simulink library "UserBlocks"  (R2014a)
settings: Solver=ode45  SolverMode=SingleTasking  StartTime=0.0  StopTime=10.0  RelTol=1e-3
values from neighbouring files (symbols this model uses):
  a = param.a    [DSC_Control_Analysis.m]    (also in DSC_Control_Analysis_Exp.m; DSC_Speed_Control_Analysis.m; EmpiricalTireCurves.m = 1.35; FFW_Fx.m = sqrt(curvature/(2*clothoidLength)))
  b = 1.15    [EmpiricalTireCurves.m]
  Cfls = Cfl    [EC_params_nissan.m]
  Crls = Crl    [EC_params_nissan.m]
  d0 = CSTR.d0    [Ext_MPCPara.m]
  freq = Fs/2*linspace(0,1,NFFT/2)    [AACplottingcode.m]    (also in If_alpha_tp_observer.m; If_alpha_tp_observer_for_c_code.m; If_alpha_tp_observer_shoreline.m)
  Iz = param.Iz    [DSC_Control_Analysis.m]    (also in DSC_Control_Analysis_Exp.m; DSC_Speed_Control_Analysis.m; EmpiricalTireCurves.m = 1300)
  K = 10    [EC_params_nissan.m]
  Ks = -10    [EC_params_nissan.m]
  Ksl = -10    [EC_params_nissan.m]
  Kt = 40000    [EC_params_nissan.m]
  Ku = -40000    [EC_params_nissan.m]
  m = 1724    [EmpiricalTireCurves.m]
  mu_s = mu_p    (= 0.6)    [EC_params_nissan.m]    (also in EmpiricalTireCurves.m = 0.55)
  Ns = 10    [EC_params_nissan.m]
  num = num+MTnum(m)    [Build_MtMuMy.m]
  q = 1    [EC_params_nissan.m]
  Taoh = CSTR.Taoh    [Ext_MPCPara.m]
  Ts = 0.002    [DSC_Control_Analysis.m]    (also in DSC_Control_Analysis_Exp.m; DSC_Speed_Control_Analysis.m; EC_params_nissan.m; Ext_MPCPara.m = SSD.Ts)
undefined symbols (not defined in the file or in its folder): acceAmp, ack, alphaFrontSteeringLimit, alphaFrontTable, bit, c, Cfl, Crl, CSTR, dden, deltaPsiDotGain, deltDist, den, denafilt, dnum, elaDotGain, filtera, filterb, frontAlphaLookup, frontForceLookup, FuelStartCalTime, FyFtable, gpsins, h, h_roll, hal_filter_den, hal_filter_num, hwx, hwy5, initAcce, initSpeed, isDriverNoise, lkparams, mapDataFull, mapMatchingParams, maxFrontForce, maxNumSegs, mdPtrs, numafilt, param, rearAlphaLookup, rfl, rfr, rrl, rrr, sglu, SIMP, simuCond, slimFxl, slimFxu, sliml, slimMll, slimMlr, slimMul, slimMur, slimu, sr, SSD, Standard, steering_limit ... (+7)
libraries: simulink x28, slrtlib x18, UserBlocks x6, slrtsoftinglib x6, MickLibBlocks x1, DriftControllerLibrary x1
(part 1 of 6)
settings Model: Creator=ddl  LastModifiedBy=cbeal

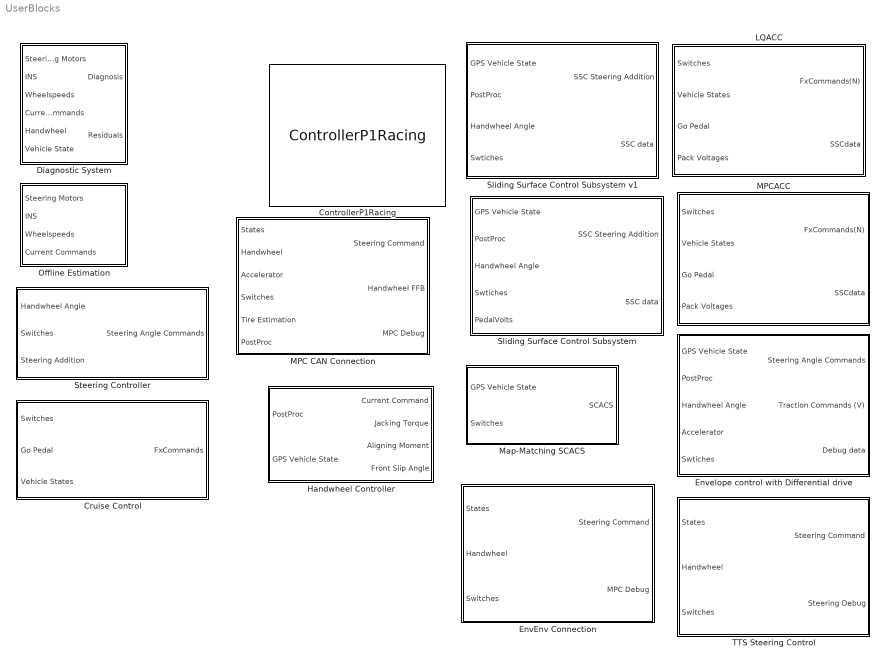
== system UserBlocks ==
  ControllerP1Racing : MickLibBlocks/ControllerP1Racing  SystemSampleTime=-1
  Cruise Control : Subsystem
      mask init:
      | CruiseControl
  Diagnostic System : Subsystem
  EnvEnv Connection : Subsystem
      mask init:
      | p1_params;
      | SteeringController;
  Envelope control with Differential drive : Subsystem
      mask init:
      | % get P1 parameters
      | p1_params;
      | 
      | % get params to filter handwheel angle
      | SteeringController;
      | 
      | Ts=0.002;
  Handwheel Controller : Subsystem
      mask init:
      | hw_lookuptable;
      | p1_params;
  LQACC : Subsystem
      mask init:
      | CruiseControl;
      | p1_params;
      | Main_MPC_MTCACC1;
  MPC CAN Connection : Subsystem
      mask init:
      | p1_params;
      | SteeringController;
  MPCACC : Subsystem
      mask init:
      | Ts = .002;
      | CruiseControl;
      | p1_params;
      | %Para_CYL52;
      | 
      | %self_ChangeDir;
      | Main_MPC_MTCACC1;
      | 
      | mpc_params;
      | LL_CtrlObj;
      | Ext_MPCpara;
      | Proc_RT_para;
  Map-Matching SCACS : Subsystem
  Offline Estimation : Subsystem
  Sliding Surface Control Subsystem : Subsystem
      mask init:
      | % get SSC parameters
      | p1_params;
      | slidingsurface_params;
      | 
      | % get params to filter handwheel angle
      | SteeringController;
  Sliding Surface Control Subsystem v1 : Subsystem
      mask init:
      | % get SSC parameters
      | p1_params;
      | slidingsurface_params;
      | 
      | % get params to filter handwheel angle
      | SteeringController;
  Steering Controller : Subsystem
      mask init:
      | p1_params;
      | SteeringController;
  TTS Steering Control : Subsystem
      mask init:
      | p1_params;
      | SteeringController;

== system UserBlocks/Cruise Control ==
  Switches : Inport
  Go Pedal : Inport  Port=2
  Vehicle States : Inport  Port=3
  Bus Selector : BusSelector  OutputSignals=Vx
  Bus Selector1 : BusSelector  OutputSignals=Cruise Control Switch,Brake Pedal Signal
  ConvertVolt2Force : Subsystem
  Enable Logic : Subsystem
  Gain : Gain
  Mux1 : Mux  Inputs=2
  Pedal Latch : Subsystem  TreatAsAtomicUnit=on
  Quantizer : Quantizer  QuantizationInterval=5
  Speed Latch : Subsystem  TreatAsAtomicUnit=on
  Sum : Sum  Inputs=-+|
  Sum1 : Sum  Inputs=|++
  Switch : Switch  Threshold=.5
  FxCommands : Outport
  wires:
  Go Pedal/1 -> Pedal Latch/1(In1), Switch/3
  Switches/1 -> Bus Selector1/1
  Sum/1 -> Gain/1
  Enable Logic/1(Enable) -> Switch/2
  Mux1/1 -> ConvertVolt2Force/1(VoltDesired)
  Switch/1 -> Mux1/2, Mux1/1
  Speed Latch/1(Out1) -> Quantizer/1
  Gain/1 -> Sum1/1
  Sum1/1 -> Switch/1
  Pedal Latch/1(Out1) -> Sum1/2
  Bus Selector1/1 -> Enable Logic/1(Cruise Control), Pedal Latch/Trigger, Speed Latch/Trigger  "<Cruise Control Switch>"
  Bus Selector1/2 -> Enable Logic/2(Brake Pedal)  "<Brake Pedal Signal>"
  Quantizer/1 -> Sum/2
  Bus Selector/1 -> Speed Latch/1(In1), Sum/1  "<Vx>"
  Vehicle States/1 -> Bus Selector/1
  ConvertVolt2Force/1(TorqueDesired) -> FxCommands/1

== system UserBlocks/Diagnostic System ==
  Steering Motors : Inport
  INS : Inport  Port=2
  Wheelspeeds : Inport  Port=3
  Current Commands : Inport  Port=4
  Handwheel : Inport  Port=5
  Vehicle State : Inport  Port=6
  Bus Selector : BusSelector  OutputSignals=Roll Angle
  Bus Selector1 : BusSelector  OutputSignals=Primary
  Bus Selector2 : BusSelector  OutputSignals=Front Wheel Speeds
  Detection : Subsystem
      mask Display: disp('')
  Filtering : Subsystem
      mask Display: disp('')
  Isolation : Subsystem
      mask Display: disp('')
  Residual Generation : Subsystem
  Diagnosis : Outport
  Residuals : Outport  Port=2
  wires:
  Steering Motors/1 -> Residual Generation/1(Steering Motors)
  INS/1 -> Residual Generation/2(INS)
  Residual Generation/1(Residuals) -> Filtering/1(Residuals)
  Detection/1(Boolean Residuals) -> Isolation/1(Boolean Residuals)
  Current Commands/1 -> Residual Generation/4(Current Commands)
  Wheelspeeds/1 -> Bus Selector2/1
  Isolation/1(Diagnosis) -> Diagnosis/1
  Filtering/1(Filtered Residuals) -> Detection/1(Filtered Residuals), Residuals/1
  Vehicle State/1 -> Bus Selector/1
  Bus Selector/1 -> Residual Generation/6(Roll Angle)  "<Roll Angle>"
  Handwheel/1 -> Bus Selector1/1
  Bus Selector1/1 -> Residual Generation/5(Handwheel)  "<Primary>"
  Bus Selector2/1 -> Residual Generation/3(Wheelspeeds)  "<Front Wheel Speeds>"

== system UserBlocks/EnvEnv Connection ==
  States : Inport
  Handwheel : Inport  Port=2
  Switches : Inport  Port=3
  Ackermann Correction : Subsystem
  Bus Selector2 : BusSelector  OutputSignals=Primary
  Bus Selector4 : BusSelector  OutputSignals=Auto-Steer Switch
  Compute delta Steer : Subsystem
  Mux6 : Mux  Inputs=2
  SW Steering Limit : Saturate  UpperLimit=steering_limit*pi/180  LowerLimit=-steering_limit*pi/180
  SW Steering Limit1 : Saturate  UpperLimit=steering_limit*pi/180  LowerLimit=-steering_limit*pi/180
  Subsystem : Subsystem
  Sum : Sum  Inputs=|++
  Sum1 : Sum  Inputs=|++
  delta offset : Constant  Value=0*pi/180
  Steering Command : Outport
  MPC Debug : Outport  Port=2
  wires:
  delta offset/1 -> Sum1/2
  Sum1/1 -> SW Steering Limit/1
  Sum/1 -> Sum1/1
  Compute delta Steer/2(MPC Debug) -> MPC Debug/1
  States/1 -> Compute delta Steer/1(States)
  Compute delta Steer/1(delta Steering Command) -> Sum/2
  SW Steering Limit1/1 -> Compute delta Steer/2(driver Steer Cmd), Sum/1
  Bus Selector4/1 -> Subsystem/2(Switches)  "<Auto-Steer Switch>"
  Bus Selector2/1 -> Subsystem/1(Handwheel)  "<Primary>"
  Switches/1 -> Compute delta Steer/3(Switches), Bus Selector4/1
  Handwheel/1 -> Bus Selector2/1
  Subsystem/1(Steering Output) -> SW Steering Limit1/1
  Ackermann Correction/2(R Steer Angle) -> Mux6/2
  Ackermann Correction/1(L Steer Angle) -> Mux6/1
  SW Steering Limit/1 -> Ackermann Correction/1(Ackermann Angle)
  Mux6/1 -> Steering Command/1

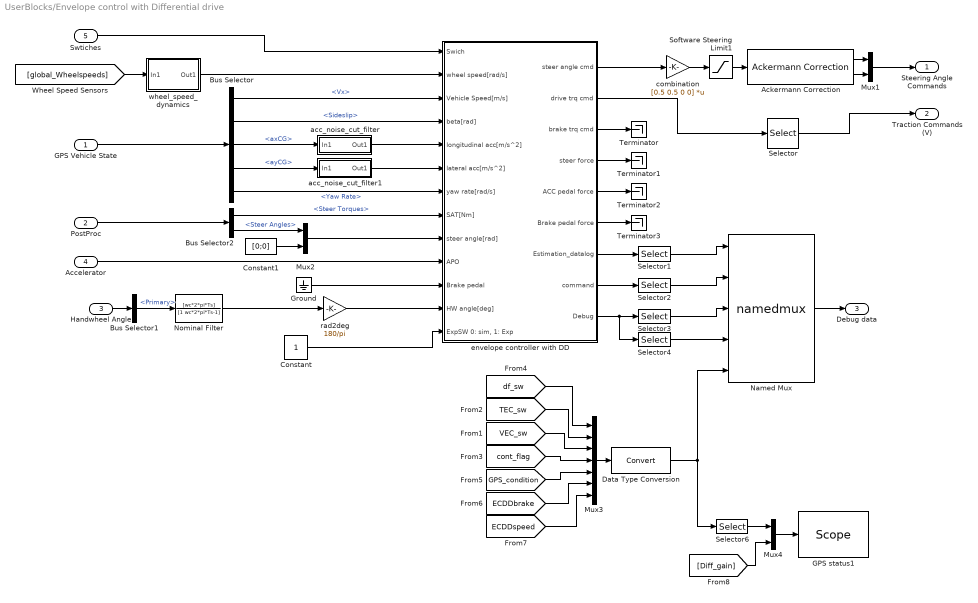
== system UserBlocks/Envelope control with Differential drive ==
  GPS Vehicle State : Inport
  PostProc : Inport  Port=2
  Handwheel Angle : Inport  Port=3
  Accelerator : Inport  Port=4
  Swtiches : Inport  Port=5
  Ackermann Correction : UserBlocks/Steering Controller/Ackermann Correction
  Bus Selector : BusSelector  OutputSignals=Vx,Sideslip,axCG,ayCG,Yaw Rate
  Bus Selector1 : BusSelector  OutputSignals=Primary
  Bus Selector2 : BusSelector  OutputSignals=Steer Torques,Steer Angles
  Constant : Constant
  Constant1 : Constant  Value=[0;0]
  Data Type Conversion : DataTypeConversion
  GPS status1 : slrtlib/Displays and Logging/Scope   scopeno=2  scopetype=Target  autostart=on  viewmode=Numerical  formatstr='%15.6f'  grid=on  ylimits=[-10,10]  nosamples=round(1/Ts)  noprepostsamples=0  interleave=1  triggermode=FreeRun  triggersignal=1  trigsignalfromport=off  triggerlevel=0.0  triggerslope=Either  triggerscope=1  triggersample=0  filename=data.dat  mode=Lazy  writesize=512  autorestart=off  dynamicfilemode=off  maxwritefilesize=512*1024^2
  Ground : Ground
  Mux1 : Mux  Inputs=2
  Mux2 : Mux  Inputs=2
  Mux3 : Mux  Inputs=7
  Mux4 : Mux  Inputs=2
  Named Mux : S-Function  FunctionName=namedmux  Parameters=inputcount,inputsizes  EnableBusSupport=off  mask{fname=datadescTCS}
      mask prompts: fname "Data description function name"
      mask help:
      | Combines input signals into a single output vector, according to a structure that provides the names and sizes of each signal.
      |
      | The parameter below should be set to the name of a function which returns a 1xN structure array, where N is the number of input signals.  The structure should contain fields "size" which specifies the width of the input signal, and "name" which specifies its name.
      mask init:
      | desc=eval(fname);
      | %if(class(desc)~='cell')
      | %	error('Incorrect description');
      | %end
      | inputcount=length(desc);
      | if((inputcount<1)|(inputcount>50))
      | 	error('Inappropriate number of inputs.');
      | end
      | 
      | inputsizes=[desc.size];
      | 
      | x=min(inputcount*ones(1,50),1:50);
      mask Display:
      | port_label('input',x(1),desc(x(1)).name);
      | port_label('input',x(2),desc(x(2)).name);
      | port_label('input',x(3),desc(x(3)).name);
      | port_label('input',x(4),desc(x(4)).name);
      | port_label('input',x(5),desc(x(5)).name);
      | port_label('input',x(6),desc(x(6)).name);
      | port_label('input',x(7),desc(x(7)).name);
      | port_label('input',x(8),desc(x(8)).name);
      | port_label('input',x(9),desc(x(9)).name);
      | port_label('input',x(10),desc(x(10)).name);
      | port_label('input',x(11),desc(x(11)).name);
      | port_label('input',x(12),desc(x(12)).name);
      | port_label('input',x(13),desc(x(13)).name);
      | port_label('input',x(14),desc(x(14)).name);
      | port_label('input',x(15),desc(x(15)).name);
      | port_label('input',x(16),desc(x(16)).name);
      | port_label('input',x(17),desc(x(17)).name);
      | port_label('input',x(18),desc(x(18)).name);
      | port_label('input',x(19),desc(x(19)).name);
      | port_label('input',x(20),desc(x(20)).name);
      | port_label('input',x(21),desc(x(21)).name);
      | port_label('input',x(22),desc(x(22)).name);
      | port_label('input',x(23),desc(x(23)).name);
      | port_label('input',x(24),desc(x(24)).name);
      | port_label('input',x(25),desc(x(25)).name);
      | port_label('input',x(26),desc(x(26)).name);
      | port_label('input',x(27),desc(x(27)).name);
      | port_label('input',x(28),desc(x(28)).name);
      | port_label('input',x(29),desc(x(29)).name);
      | port_label('input',x(30),desc(x(30)).name);
  Nominal Filter : DiscreteFilter  Numerator=[wc*2*pi*Ts]  Denominator=[1 wc*2*pi*Ts-1]  SampleTime=Ts
  Selector : Selector  InputPortWidth=4  Indices=[4 3]
  Selector1 : Selector  InputPortWidth=17  Indices=[1:4]
  Selector2 : Selector  InputPortWidth=9  Indices=[7:9]
  Selector3 : Selector  InputPortWidth=19  Indices=[1:8]
  Selector4 : Selector  InputPortWidth=19  Indices=[9,11:19]
  Selector6 : Selector  InputPortWidth=7  Indices=[4:7]
  Software Steering Limit1 : Saturate  UpperLimit=steering_limit*pi/180  LowerLimit=-steering_limit*pi/180
  Terminator{,1..3} (4 alike) : Terminator
  acc_noise_cut_filter : Subsystem
      mask init:
      | [numafilt,denafilt]=butter(2,0.02);
  acc_noise_cut_filter1 : Subsystem
      mask init:
      | [numafilt,denafilt]=butter(2,0.02);
  combination : Gain  Gain=[0.5 0.5 0 0]  Multiplication=Matrix(K*u)
  envelope controller with DD : Subsystem
      mask init:
      | p1_params
  rad2deg : Gain  Gain=180/pi
  wheel_speed_dynamics : Subsystem
      mask init:
      | p1_params
      | EC_params_nissan
      | [filterb,filtera]=butter(2,0.03);
  Steering Angle Commands : Outport
  Traction Commands (V) : Outport  Port=2
  Debug data : Outport  Port=3
  wires:
  [Diff_gain] -> Mux4/2
  Mux4/1 -> GPS status1/1
  Selector6/1 -> Mux4/1
  [ECDDspeed] -> Mux3/7
  [ECDDbrake] -> Mux3/6
  [GPS_condition] -> Mux3/5
  [cont_flag] -> Mux3/4
  [VEC_sw] -> Mux3/3
  [TEC_sw] -> Mux3/2
  [df_sw] -> Mux3/1
  Selector4/1 -> Named Mux/4
  acc_noise_cut_filter1/1(Out1) -> envelope controller with DD/6(lateral acc[m/s^2])
  acc_noise_cut_filter/1(Out1) -> envelope controller with DD/5(longitudinal acc[m/s^2])
  Data Type Conversion/1 -> Named Mux/5, Selector6/1
  Handwheel Angle/1 -> Bus Selector1/1
  Ground/1 -> envelope controller with DD/11(Brake pedal)
  Mux2/1 -> envelope controller with DD/9(steer angle[rad])
  Software Steering Limit1/1 -> Ackermann Correction/1
  Ackermann Correction/1 -> Mux1/1
  Ackermann Correction/2 -> Mux1/2
  Mux1/1 -> Steering Angle Commands/1
  combination/1 -> Software Steering Limit1/1
  Selector/1 -> Traction Commands (V)/1
  envelope controller with DD/3(brake trq cmd) -> Terminator/1
  envelope controller with DD/4(steer force) -> Terminator1/1
  envelope controller with DD/5(ACC pedal force) -> Terminator2/1
  envelope controller with DD/6(Brake pedal force) -> Terminator3/1
  envelope controller with DD/7(Estimation_datalog) -> Selector1/1
  envelope controller with DD/2(drive trq cmd) -> Selector/1
  envelope controller with DD/8(command) -> Selector2/1
  envelope controller with DD/9(Debug) -> Selector3/1, Selector4/1
  Selector1/1 -> Named Mux/1
  Selector2/1 -> Named Mux/2
  Selector3/1 -> Named Mux/3
  Named Mux/1 -> Debug data/1
  Bus Selector1/1 -> Nominal Filter/1  "<Primary>"
  Nominal Filter/1 -> rad2deg/1
  rad2deg/1 -> envelope controller with DD/12(HW angle[deg])
  Constant/1 -> envelope controller with DD/13("ExpSW 0: sim, 1: Exp")
  GPS Vehicle State/1 -> Bus Selector/1
  PostProc/1 -> Bus Selector2/1
  Bus Selector2/1 -> envelope controller with DD/8(SAT[Nm])  "<Steer Torques>"
  Bus Selector2/2 -> Mux2/1  "<Steer Angles>"
  Constant1/1 -> Mux2/2
  Accelerator/1 -> envelope controller with DD/10(APO)
  Bus Selector/1 -> envelope controller with DD/3(Vehicle Speed[m/s])  "<Vx>"
  Bus Selector/5 -> envelope controller with DD/7(yaw rate[rad/s])  "<Yaw Rate>"
  Bus Selector/2 -> envelope controller with DD/4(beta[rad])  "<Sideslip>"
  Bus Selector/3 -> acc_noise_cut_filter/1(In1)  "<axCG>"
  Bus Selector/4 -> acc_noise_cut_filter1/1(In1)  "<ayCG>"
  wheel_speed_dynamics/1(Out1) -> envelope controller with DD/2(wheel speed[rad/s])
  [global_Wheelspeeds] -> wheel_speed_dynamics/1(In1)
  envelope controller with DD/1(steer angle cmd) -> combination/1
  Swtiches/1 -> envelope controller with DD/1(Swich)
  Mux3/1 -> Data Type Conversion/1

== system UserBlocks/Handwheel Controller ==
  note: alpha slide
  note: Fy
  note: pneumatic trail
  note: Simulated Aligning Moment Cmd, max=.7
  note: Simulated Jacking Torque Cmd, max=.25
  note: avg steer angle
  PostProc : Inport
  GPS Vehicle State : Inport  Port=2
  Bus Selector2 : BusSelector  OutputSignals=Composite Steer Angle
  Bus Selector3 : BusSelector  OutputSignals=Vx,Yaw Rate,VyCG
  Gain1 : Gain  Gain=100
  Gain2 : Gain  Gain=1/125
  Gain3 : Gain  Gain=.0008
  Sum : Sum  Inputs=+|+
  T4 : Terminator
  T6 : Terminator
  T7 : Terminator
  estimate_aligningTorque : S-Function  FunctionName=estimate_aligningTorque  Parameters=tp, Cf, Fz_f, tm, b  EnableBusSupport=off
  jacking torque cmd with 0.25 saturation : Lookup  InputValues=hwx.*100  Table=hwy5.*100  OutDataTypeStr=float('double')  SaturateOnIntegerOverflow=on
  Current Command : Outport
  Jacking Torque : Outport  Port=2
  Aligning Moment : Outport  Port=3
  Front Slip Angle : Outport  Port=4
  wires:
  estimate_aligningTorque/5 -> Front Slip Angle/1  "alpha_f"
  Bus Selector3/3 -> estimate_aligningTorque/4  "<VyCG>"
  Bus Selector3/2 -> estimate_aligningTorque/3  "<Yaw Rate>"
  Bus Selector3/1 -> estimate_aligningTorque/2  "<Vx>"
  GPS Vehicle State/1 -> Bus Selector3/1
  Sum/1 -> Current Command/1
  Gain3/1 -> Aligning Moment/1, Sum/2  "Align Mom Cmd"
  estimate_aligningTorque/1 -> Gain3/1
  estimate_aligningTorque/4 -> T7/1
  estimate_aligningTorque/3 -> T6/1
  estimate_aligningTorque/2 -> T4/1
  Bus Selector2/1 -> estimate_aligningTorque/1, Gain1/1  "<Composite Steer Angle>"
  Gain2/1 -> Jacking Torque/1, Sum/1  "Jack Torque Cmd"
  jacking torque cmd with 0.25 saturation/1 -> Gain2/1
  Gain1/1 -> jacking torque cmd with 0.25 saturation/1
  PostProc/1 -> Bus Selector2/1

== system UserBlocks/LQACC ==
  Switches : Inport
  Vehicle States : Inport  Port=2
  Go Pedal : Inport  Port=3
  Pack Voltages : Inport  Port=4
  Bus Creator : BusCreator  Inputs=10
  Bus Selector : BusSelector  OutputSignals=Traction
  PIDACC : Subsystem  AncestorBlock=UserBlocks/Cruise Control
      mask init:
      | CruiseControl;
      | p1_params;
      | Main_MPC_MTCACC1;
  FxCommands(N) : Outport
  SSCdata : Outport  Port=2
  wires:
  PIDACC/10(vehACCE) -> Bus Creator/10
  PIDACC/9(relVEL) -> Bus Creator/9
  PIDACC/8(distErr) -> Bus Creator/8
  PIDACC/7(desAcce(m/s2)) -> Bus Creator/6
  Pack Voltages/1 -> Bus Selector/1
  Bus Creator/1 -> SSCdata/1
  Switches/1 -> PIDACC/1(Switches)
  Vehicle States/1 -> PIDACC/2(Vehicle States)
  Go Pedal/1 -> PIDACC/3(Go Pedal1)
  Bus Selector/1 -> Bus Creator/7  "<Traction>"
  PIDACC/1(FxCommands(N)) -> FxCommands(N)/1
  PIDACC/2(PreAcce(m/s2)) -> Bus Creator/1
  PIDACC/3(PreSpeec(m/s)) -> Bus Creator/2
  PIDACC/4(epsilon) -> Bus Creator/3
  PIDACC/5(DesDist(m)) -> Bus Creator/4
  PIDACC/6(ActDist(m)) -> Bus Creator/5

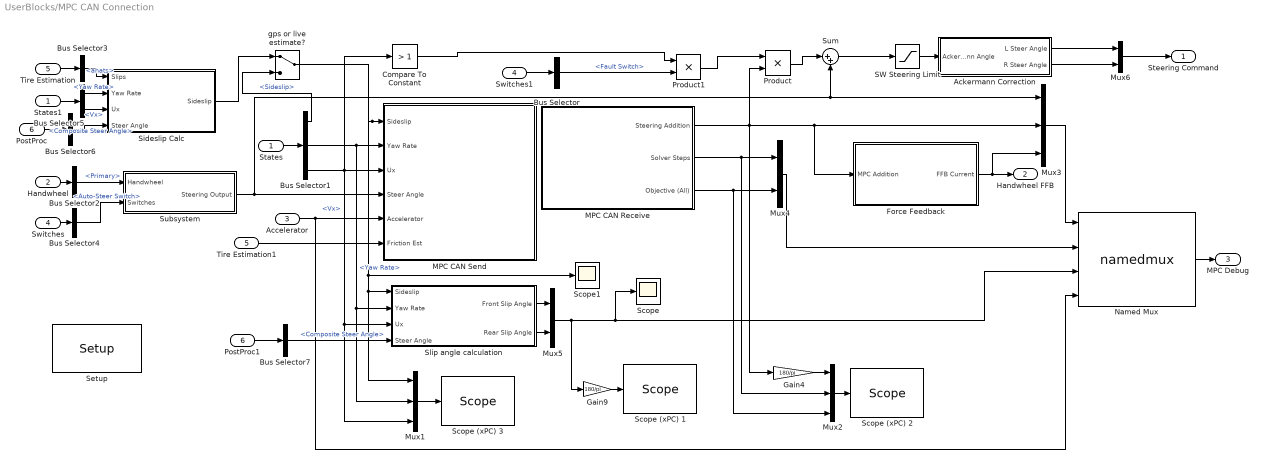
== system UserBlocks/MPC CAN Connection ==
  States : Inport
  Handwheel : Inport  Port=2
  Accelerator : Inport  Port=3
  Switches : Inport  Port=4
  Tire Estimation : Inport  Port=5
  PostProc : Inport  Port=6
  Ackermann Correction : Subsystem
  Bus Selector : BusSelector  OutputSignals=Fault Switch
  Bus Selector1 : BusSelector  OutputSignals=Sideslip,Yaw Rate,Vx
  Bus Selector2 : BusSelector  OutputSignals=Primary
  Bus Selector3 : BusSelector  OutputSignals=ahats
  Bus Selector4 : BusSelector  OutputSignals=Auto-Steer Switch
  Bus Selector5 : BusSelector  OutputSignals=Yaw Rate,Vx
  Bus Selector6 : BusSelector  OutputSignals=Composite Steer Angle
  Bus Selector7 : BusSelector  OutputSignals=Composite Steer Angle
  Compare To Constant : simulink/Logic and Bit Operations/Compare To Constant  relop=>  const=1  OutDataTypeStr=uint8  ZeroCross=off
  Force Feedback : Subsystem  mask{steer_gain=0, current_limit=0}
      mask prompts: steer_gain "FFB Gain (A/rad)"; current_limit "Current Limit (A)"
  Gain4 : Gain  Gain=180/pi
  Gain9 : Gain  Gain=180/pi
  MPC CAN Receive : Subsystem
  MPC CAN Send : Subsystem
  Mux1 : Mux  Inputs=3
  Mux2 : Mux  Inputs=3
  Mux3 : Mux  Inputs=3
  Mux4 : Mux  Inputs=2
  Mux5 : Mux  Inputs=2
  Mux6 : Mux  Inputs=2
  Named Mux : S-Function  FunctionName=namedmux  Parameters=inputcount,inputsizes  EnableBusSupport=off  mask{fname=datadescMPCEnv}
      mask prompts: fname "Data description function name"
      mask help:
      | Combines input signals into a single output vector, according to a structure that provides the names and sizes of each signal.
      |
      | The parameter below should be set to the name of a function which returns a 1xN structure array, where N is the number of input signals.  The structure should contain fields "size" which specifies the width of the input signal, and "name" which specifies its name.
      mask init: same as UserBlocks/Envelope control with Differential drive/Named Mux
      mask Display:
      | port_label('input',x(1),desc(x(1)).name);
      | port_label('input',x(2),desc(x(2)).name);
      | port_label('input',x(3),desc(x(3)).name);
      | port_label('input',x(4),desc(x(4)).name);
      | port_label('input',x(5),desc(x(5)).name);
      | port_label('input',x(6),desc(x(6)).name);
      | port_label('input',x(7),desc(x(7)).name);
      | port_label('input',x(8),desc(x(8)).name);
      | port_label('input',x(9),desc(x(9)).name);
      | port_label('input',x(10),desc(x(10)).name);
      | port_label('input',x(11),desc(x(11)).name);
      | port_label('input',x(12),desc(x(12)).name);
      | port_label('input',x(13),desc(x(13)).name);
      | port_label('input',x(14),desc(x(14)).name);
      | port_label('input',x(15),desc(x(15)).name);
      | port_label('input',x(16),desc(x(16)).name);
      | port_label('input',x(17),desc(x(17)).name);
      | port_label('input',x(18),desc(x(18)).name);
      | port_label('input',x(19),desc(x(19)).name);
      | port_label('input',x(20),desc(x(20)).name);
      | port_label('input',x(21),desc(x(21)).name);
      | port_label('input',x(22),desc(x(22)).name);
      | port_label('input',x(23),desc(x(23)).name);
      | port_label('input',x(24),desc(x(24)).name);
      | port_label('input',x(25),desc(x(25)).name);
      | port_label('input',x(26),desc(x(26)).name);
      | port_label('input',x(27),desc(x(27)).name);
      | port_label('input',x(28),desc(x(28)).name);
      | port_label('input',x(29),desc(x(29)).name);
      | port_label('input',x(30),desc(x(30)).name);
  PostProc1 : InportShadow  Port=6
  Product : Product  RndMeth=Zero
  Product1 : Product  RndMeth=Zero
  SW Steering Limit : Saturate  UpperLimit=steering_limit*pi/180  LowerLimit=-steering_limit*pi/180
  Scope : Scope
  Scope (xPC) 1 : slrtlib/Displays and Logging/Scope   scopeno=3  scopetype=Target  autostart=on  viewmode=Graphical rolling  formatstr='%15.6f'  grid=on  ylimits=[-10,10]  nosamples=50  noprepostsamples=0  interleave=1  triggermode=FreeRun  triggersignal=1  trigsignalfromport=off  triggerlevel=0.0  triggerslope=Either  triggerscope=1  triggersample=0  filename=data.dat  mode=Lazy  writesize=512  autorestart=off  dynamicfilemode=off  maxwritefilesize=512*1024^2
  Scope (xPC) 2 : slrtlib/Displays and Logging/Scope   scopeno=4  scopetype=Target  autostart=on  viewmode=Numerical  formatstr='%15.6f'  grid=on  ylimits=[-1,1]  nosamples=100  noprepostsamples=0  interleave=1  triggermode=FreeRun  triggersignal=1  trigsignalfromport=off  triggerlevel=0.0  triggerslope=Either  triggerscope=1  triggersample=0  filename=data.dat  mode=Lazy  writesize=512  autorestart=off  dynamicfilemode=off  maxwritefilesize=512*1024^2
  Scope (xPC) 3 : slrtlib/Displays and Logging/Scope   scopeno=2  scopetype=Target  autostart=on  viewmode=Numerical  formatstr='%15.6f'  grid=on  ylimits=[-30,30]  nosamples=50  noprepostsamples=0  interleave=1  triggermode=FreeRun  triggersignal=1  trigsignalfromport=off  triggerlevel=0.0  triggerslope=Either  triggerscope=1  triggersample=0  filename=data.dat  mode=Lazy  writesize=512  autorestart=off  dynamicfilemode=off  maxwritefilesize=512*1024^2
  Scope1 : Scope
  "Setup " : slrtsoftinglib/CAN-AC2-104 SJA 1000/Setup   board=1  can1Baudrate=500 kBaud  can1UserBR=[1,1,4,3]  can2Baudrate=500 kBaud  can2UserBR=[1,1,4,3]  init=[]  term=[]  bus_off_out=off  bus_off_rec=Off  ioBaseAddressL=0x240  memBaseAddressL=0xd0000  intNo=None
  Sideslip Calc : Subsystem  mask{a=1.35, b=1.15}
      mask prompts: a "CG - Front Axle Distance"; b "CG - Rear Axle Distance"
  Slip angle calculation : Subsystem  mask{a=1.35, b=1.15}
      mask prompts: a "CG - Front Axle Distance"; b "CG - Rear Axle Distance"
  States1 : InportShadow
  Subsystem : Subsystem
  Sum : Sum  Inputs=|++
  Switches1 : InportShadow  Port=4
  Tire Estimation1 : InportShadow  Port=5
  gps or live estimate? : ManualSwitch
  Steering Command : Outport
  Handwheel FFB : Outport  Port=2
  MPC Debug : Outport  Port=3
  wires:
  Bus Selector7/1 -> Slip angle calculation/4(Steer Angle)  "<Composite Steer Angle>"
  PostProc1/1 -> Bus Selector7/1
  Bus Selector6/1 -> Sideslip Calc/4(Steer Angle)  "<Composite Steer Angle>"
  PostProc/1 -> Bus Selector6/1
  Bus Selector1/1 -> gps or live estimate?/2  "<Sideslip>"
  gps or live estimate?/1 -> Mux1/1, Slip angle calculation/1(Sideslip), Scope1/1, MPC CAN Send/1(Sideslip)
  Sideslip Calc/1(Sideslip) -> gps or live estimate?/1
  Tire Estimation1/1 -> MPC CAN Send/6(Friction Est)
  Bus Selector5/2 -> Sideslip Calc/3(Ux)  "<Vx>"
  Bus Selector5/1 -> Sideslip Calc/2(Yaw Rate)  "<Yaw Rate>"
  Bus Selector3/1 -> Sideslip Calc/1(Slips)  "<ahats>"
  States1/1 -> Bus Selector5/1
  Tire Estimation/1 -> Bus Selector3/1
  Mux6/1 -> Steering Command/1
  Product1/1 -> Product/1
  Compare To Constant/1 -> Product1/1
  Bus Selector/1 -> Product1/2  "<Fault Switch>"
  Switches1/1 -> Bus Selector/1
  SW Steering Limit/1 -> Ackermann Correction/1(Ackermann Angle)
  Ackermann Correction/1(L Steer Angle) -> Mux6/1
  Ackermann Correction/2(R Steer Angle) -> Mux6/2
  Named Mux/1 -> MPC Debug/1
  Mux5/1 -> Scope/1, Named Mux/3, Gain9/1
  Mux4/1 -> Named Mux/2
  Slip angle calculation/2(Rear Slip Angle) -> Mux5/2
  Slip angle calculation/1(Front Slip Angle) -> Mux5/1
  Gain4/1 -> Mux2/1
  Mux2/1 -> Scope (xPC) 2/1
  States/1 -> Bus Selector1/1
  Bus Selector1/3 -> MPC CAN Send/3(Ux), Slip angle calculation/3(Ux), Mux1/3, Compare To Constant/1  "<Vx>"
  Mux3/1 -> Named Mux/1
  MPC CAN Receive/1(Steering Addition) -> Force Feedback/1(MPC Addition), Mux3/2, Gain4/1, Product/2
  Sum/1 -> SW Steering Limit/1
  Force Feedback/1(FFB Current) -> Handwheel FFB/1, Mux3/3
  Bus Selector1/2 -> MPC CAN Send/2(Yaw Rate), Slip angle calculation/2(Yaw Rate), Mux1/2  "<Yaw Rate>"
  MPC CAN Receive/2(Solver Steps) -> Mux4/1, Mux2/2
  MPC CAN Receive/3(Objective (All)) -> Mux4/2, Mux2/3
  Gain9/1 -> Scope (xPC) 1/1
  Mux1/1 -> Scope (xPC) 3/1
  Accelerator/1 -> Named Mux/4, MPC CAN Send/5(Accelerator)
  Product/1 -> Sum/1
  Subsystem/1(Steering Output) -> Mux3/1, Sum/2, MPC CAN Send/4(Steer Angle)
  Handwheel/1 -> Bus Selector2/1
  Switches/1 -> Bus Selector4/1
  Bus Selector2/1 -> Subsystem/1(Handwheel)  "<Primary>"
  Bus Selector4/1 -> Subsystem/2(Switches)  "<Auto-Steer Switch>"

== system UserBlocks/MPCACC ==
  Switches : Inport
  Vehicle States : Inport  Port=2
  Go Pedal : Inport  Port=3
  Pack Voltages : Inport  Port=4
  Bus Creator : BusCreator  Inputs=10
  Bus Selector : BusSelector  OutputSignals=Traction
  PIDACC : Subsystem  AncestorBlock=UserBlocks/Cruise Control
      mask init:
      | InitModel;
      | CruiseControl;
      | p1_params;
      | Main_MPC_MTCACC1;
  FxCommands(N) : Outport
  SSCdata : Outport  Port=2
  wires:
  PIDACC/6(ActDist(m)) -> Bus Creator/5
  PIDACC/5(DesDist(m)) -> Bus Creator/4
  PIDACC/4(epsilon) -> Bus Creator/3
  PIDACC/3(PreSpeec(m/s)) -> Bus Creator/2
  PIDACC/2(PreAcce(m/s2)) -> Bus Creator/1
  PIDACC/1(FxCommands(N)) -> FxCommands(N)/1
  Bus Selector/1 -> Bus Creator/7  "<Traction>"
  Go Pedal/1 -> PIDACC/3(Go Pedal1)
  Vehicle States/1 -> PIDACC/2(Vehicle States)
  Switches/1 -> PIDACC/1(Switches)
  Bus Creator/1 -> SSCdata/1
  Pack Voltages/1 -> Bus Selector/1
  PIDACC/7(desAcce(m/s2)) -> Bus Creator/6
  PIDACC/8(distErr) -> Bus Creator/8
  PIDACC/9(relVEL) -> Bus Creator/9
  PIDACC/10(vehACCE) -> Bus Creator/10

== system UserBlocks/Map-Matching SCACS ==
  GPS Vehicle State : Inport
  Switches : Inport  Port=2
  Bus Creator : BusCreator  Inputs=6
  Bus Selector : BusSelector  OutputSignals=Pos E,Pos N,Yaw Angle,Vx
  Bus Selector1 : BusSelector  OutputSignals=Auto-Steer Switch
  Constant1 : Constant  Value=pi/2  SampleTime=Ts
  SCACS Map-Matching : Subsystem
  Sum : Sum  Inputs=|++
  initSeg : Constant  Value=0
  SCACS : Outport
  wires:
  Bus Selector/4 -> SCACS Map-Matching/4(vx_cg)  "<Vx>"
  initSeg/1 -> SCACS Map-Matching/6(initSeg)
  SCACS Map-Matching/5(debugOut) -> Bus Creator/5  "debugOut"
  SCACS Map-Matching/4(twoOut) -> Bus Creator/4  "twoOut"
  SCACS Map-Matching/3(nextOut) -> Bus Creator/3  "nextOut"
  SCACS Map-Matching/2(currentOut) -> Bus Creator/2  "currentOut"
  SCACS Map-Matching/1(matchOut) -> Bus Creator/1  "matchOut"
  Bus Selector1/1 -> SCACS Map-Matching/5(enable)  "<Auto-Steer Switch>"
  GPS Vehicle State/1 -> Bus Selector/1
  Bus Selector/1 -> SCACS Map-Matching/1(positionEast)  "<Pos E>"
  Bus Selector/2 -> SCACS Map-Matching/2(positionNorth)  "<Pos N>"
  Bus Creator/1 -> SCACS/1
  Bus Selector/3 -> Sum/1  "<Yaw Angle>"
  Sum/1 -> SCACS Map-Matching/3(yawAngle)
  Constant1/1 -> Sum/2
  Switches/1 -> Bus Selector1/1
  SCACS Map-Matching/6(thrOut) -> Bus Creator/6  "thrOut"

== system UserBlocks/Offline Estimation ==
  note: Hook diagnostic or estimator blocks to either the
      | unfaulted or faulted signals as necessary...
  Steering Motors : Inport
  INS : Inport  Port=2
  Wheelspeeds : Inport  Port=3
  Current Commands : Inport  Port=4
  Bus Selector : BusSelector  OutputSignals=Front Wheel Speeds
  Data Extractor : Subsystem
      mask init:
      | [filterb,filtera]=butter(5,0.02);
      | InitModel;
      | ssest_params;
      | p1_params;
      | nissan_steer_lookup_data;
  Fault Maker : Subsystem
      mask init:
      | [filterb,filtera]=butter(5,0.02);
  Mux : Mux
  Terminator : Terminator
  wires:
  Steering Motors/1 -> Data Extractor/1(Steering Motors)
  INS/1 -> Data Extractor/2(INS)
  Current Commands/1 -> Data Extractor/4(Current Commands)
  Wheelspeeds/1 -> Bus Selector/1
  Data Extractor/1(Steer Angles) -> Mux/1
  Data Extractor/2(Motor Currents) -> Mux/2
  Data Extractor/3(Yaw Rate) -> Mux/3
  Data Extractor/4(Velocity) -> Mux/4
  Mux/1 -> Fault Maker/1(Unfaulted)
  Fault Maker/1(Faulted) -> Terminator/1
  Bus Selector/1 -> Data Extractor/3(Wheelspeeds)  "<Front Wheel Speeds>"

== system UserBlocks/Sliding Surface Control Subsystem ==
  GPS Vehicle State : Inport
  PostProc : Inport  Port=2
  Handwheel Angle : Inport  Port=3
  Swtiches : Inport  Port=4
  PedalVolts : Inport  Port=5
  Bus Selector : BusSelector  OutputSignals=Sideslip,Yaw Rate,Vx
  Bus Selector1 : BusSelector  OutputSignals=Composite Steer Angle
  Bus Selector2 : BusSelector  OutputSignals=Fault Switch
  Bus Selector3 : BusSelector  OutputSignals=Primary
  Mux : Mux  Inputs=14
  Named Mux : S-Function  FunctionName=namedmux  Parameters=inputcount,inputsizes  EnableBusSupport=off  mask{fname=datadescSSC}
      mask prompts: fname "Data description function name"
      mask help:
      | Combines input signals into a single output vector, according to a structure that provides the names and sizes of each signal.
      |
      | The parameter below should be set to the name of a function which returns a 1xN structure array, where N is the number of input signals.  The structure should contain fields "size" which specifies the width of the input signal, and "name" which specifies its name.
      mask init: same as UserBlocks/Envelope control with Differential drive/Named Mux
      mask Display:
      | port_label('input',x(1),desc(x(1)).name);
      | port_label('input',x(2),desc(x(2)).name);
      | port_label('input',x(3),desc(x(3)).name);
      | port_label('input',x(4),desc(x(4)).name);
      | port_label('input',x(5),desc(x(5)).name);
      | port_label('input',x(6),desc(x(6)).name);
      | port_label('input',x(7),desc(x(7)).name);
      | port_label('input',x(8),desc(x(8)).name);
      | port_label('input',x(9),desc(x(9)).name);
      | port_label('input',x(10),desc(x(10)).name);
      | port_label('input',x(11),desc(x(11)).name);
      | port_label('input',x(12),desc(x(12)).name);
      | port_label('input',x(13),desc(x(13)).name);
      | port_label('input',x(14),desc(x(14)).name);
      | port_label('input',x(15),desc(x(15)).name);
      | port_label('input',x(16),desc(x(16)).name);
      | port_label('input',x(17),desc(x(17)).name);
      | port_label('input',x(18),desc(x(18)).name);
      | port_label('input',x(19),desc(x(19)).name);
      | port_label('input',x(20),desc(x(20)).name);
      | port_label('input',x(21),desc(x(21)).name);
      | port_label('input',x(22),desc(x(22)).name);
      | port_label('input',x(23),desc(x(23)).name);
      | port_label('input',x(24),desc(x(24)).name);
      | port_label('input',x(25),desc(x(25)).name);
      | port_label('input',x(26),desc(x(26)).name);
      | port_label('input',x(27),desc(x(27)).name);
      | port_label('input',x(28),desc(x(28)).name);
      | port_label('input',x(29),desc(x(29)).name);
      | port_label('input',x(30),desc(x(30)).name);
  Nominal Filter : DiscreteFilter  Numerator=[wc*2*pi*Ts]  Denominator=[1 wc*2*pi*Ts-1]  SampleTime=Ts
  Sliding Surface Controller function : Subsystem
      mask init:
      | p1_params;
      | slidingsurface_params;
  Software Steering Limit : Saturate  UpperLimit=steering_limit*pi/180  LowerLimit=-steering_limit*pi/180
  Steering Ratio : Gain  Gain=1/sr  SaturateOnIntegerOverflow=on  OutDataTypeStr=Inherit: Same as input  ParamDataTypeStr=Inherit: Same as input
  SSC Steering Addition : Outport
  SSC data : Outport  Port=2
  wires:
  Sliding Surface Controller function/15(EnableIncontrol) -> Mux/14
  Sliding Surface Controller function/14(d_incontrol) -> Mux/13
  Sliding Surface Controller function/13(incontrol_angle) -> Mux/12
  Sliding Surface Controller function/12(incontrol_maxangle) -> Mux/11
  PedalVolts/1 -> Sliding Surface Controller function/7(Pedal)
  Bus Selector2/1 -> Sliding Surface Controller function/6(Enable)  "<Fault Switch>"
  Mux/1 -> Named Mux/2
  Bus Selector1/1 -> Sliding Surface Controller function/5(d)  "<Composite Steer Angle>"
  Software Steering Limit/1 -> Sliding Surface Controller function/4(Handwheel)
  PostProc/1 -> Bus Selector1/1
  GPS Vehicle State/1 -> Bus Selector/1
  Handwheel Angle/1 -> Bus Selector3/1
  Bus Selector3/1 -> Nominal Filter/1  "<Primary>"
  Nominal Filter/1 -> Steering Ratio/1
  Steering Ratio/1 -> Software Steering Limit/1
  Bus Selector/1 -> Sliding Surface Controller function/1(B)  "<Sideslip>"
  Bus Selector/2 -> Sliding Surface Controller function/2(r)  "<Yaw Rate>"
  Bus Selector/3 -> Sliding Surface Controller function/3(Vx)  "<Vx>"
  Swtiches/1 -> Bus Selector2/1
  Named Mux/1 -> SSC data/1
  Sliding Surface Controller function/10(EnableControl) -> Mux/9
  Sliding Surface Controller function/1(d_addition) -> SSC Steering Addition/1, Named Mux/1
  Sliding Surface Controller function/2(d_control) -> Mux/1
  Sliding Surface Controller function/3(S) -> Mux/2
  Sliding Surface Controller function/4(rsafe) -> Mux/3
  Sliding Surface Controller function/5(Bsafe) -> Mux/4
  Sliding Surface Controller function/6(rsafe_dot) -> Mux/5
  Sliding Surface Controller function/7(Bsafe_dot) -> Mux/6
  Sliding Surface Controller function/8(Fyf_control) -> Mux/7
  Sliding Surface Controller function/9(Fyr) -> Mux/8
  Sliding Surface Controller function/11(delta_dot) -> Mux/10

== system UserBlocks/Sliding Surface Control Subsystem v1 ==
  GPS Vehicle State : Inport
  PostProc : Inport  Port=2
  Handwheel Angle : Inport  Port=3
  Swtiches : Inport  Port=4
  Bus Selector : BusSelector  OutputSignals=Sideslip,Yaw Rate,Vx
  Bus Selector1 : BusSelector  OutputSignals=Composite Steer Angle
  Bus Selector2 : BusSelector  OutputSignals=Fault Switch
  Bus Selector3 : BusSelector  OutputSignals=Primary
  Mux : Mux  Inputs=10
  Named Mux : S-Function  FunctionName=namedmux  Parameters=inputcount,inputsizes  EnableBusSupport=off  mask{fname=datadescSSC}
      mask prompts: fname "Data description function name"
      mask help:
      | Combines input signals into a single output vector, according to a structure that provides the names and sizes of each signal.
      |
      | The parameter below should be set to the name of a function which returns a 1xN structure array, where N is the number of input signals.  The structure should contain fields "size" which specifies the width of the input signal, and "name" which specifies its name.
      mask init: same as UserBlocks/Envelope control with Differential drive/Named Mux
      mask Display:
      | port_label('input',x(1),desc(x(1)).name);
      | port_label('input',x(2),desc(x(2)).name);
      | port_label('input',x(3),desc(x(3)).name);
      | port_label('input',x(4),desc(x(4)).name);
      | port_label('input',x(5),desc(x(5)).name);
      | port_label('input',x(6),desc(x(6)).name);
      | port_label('input',x(7),desc(x(7)).name);
      | port_label('input',x(8),desc(x(8)).name);
      | port_label('input',x(9),desc(x(9)).name);
      | port_label('input',x(10),desc(x(10)).name);
      | port_label('input',x(11),desc(x(11)).name);
      | port_label('input',x(12),desc(x(12)).name);
      | port_label('input',x(13),desc(x(13)).name);
      | port_label('input',x(14),desc(x(14)).name);
      | port_label('input',x(15),desc(x(15)).name);
      | port_label('input',x(16),desc(x(16)).name);
      | port_label('input',x(17),desc(x(17)).name);
      | port_label('input',x(18),desc(x(18)).name);
      | port_label('input',x(19),desc(x(19)).name);
      | port_label('input',x(20),desc(x(20)).name);
      | port_label('input',x(21),desc(x(21)).name);
      | port_label('input',x(22),desc(x(22)).name);
      | port_label('input',x(23),desc(x(23)).name);
      | port_label('input',x(24),desc(x(24)).name);
      | port_label('input',x(25),desc(x(25)).name);
      | port_label('input',x(26),desc(x(26)).name);
      | port_label('input',x(27),desc(x(27)).name);
      | port_label('input',x(28),desc(x(28)).name);
      | port_label('input',x(29),desc(x(29)).name);
      | port_label('input',x(30),desc(x(30)).name);
  Nominal Filter : DiscreteFilter  Numerator=[wc*2*pi*Ts]  Denominator=[1 wc*2*pi*Ts-1]  SampleTime=Ts
  Sliding Surface Controller function : Subsystem
      mask init:
      | p1_params;
      | slidingsurface_params;
  Software Steering Limit : Saturate  UpperLimit=steering_limit*pi/180  LowerLimit=-steering_limit*pi/180
  Steering Ratio : Gain  Gain=1/sr  SaturateOnIntegerOverflow=on  OutDataTypeStr=Inherit: Same as input  ParamDataTypeStr=Inherit: Same as input
  SSC Steering Addition : Outport
  SSC data : Outport  Port=2
  wires:
  Named Mux/1 -> SSC data/1
  Sliding Surface Controller function/10(EnableControl) -> Mux/9
  Bus Selector2/1 -> Sliding Surface Controller function/4(Enable)  "<Fault Switch>"
  Swtiches/1 -> Bus Selector2/1
  Sliding Surface Controller function/5(Bnom) -> Mux/4
  Sliding Surface Controller function/2(d_control) -> Mux/1
  Sliding Surface Controller function/3(S) -> Mux/2
  Sliding Surface Controller function/4(rnom) -> Mux/3
  Sliding Surface Controller function/6(rnom_dot) -> Mux/5
  Sliding Surface Controller function/7(Bnom_dot) -> Mux/6
  Sliding Surface Controller function/8(Fyf_control) -> Mux/7
  Sliding Surface Controller function/9(Fyr) -> Mux/8
  Bus Selector/3 -> Sliding Surface Controller function/3(Vx)  "<Vx>"
  Bus Selector/2 -> Sliding Surface Controller function/2(r)  "<Yaw Rate>"
  Bus Selector/1 -> Sliding Surface Controller function/1(B)  "<Sideslip>"
  Sliding Surface Controller function/1(d_addition) -> SSC Steering Addition/1, Named Mux/1
  Steering Ratio/1 -> Software Steering Limit/1
  Nominal Filter/1 -> Steering Ratio/1
  Bus Selector3/1 -> Nominal Filter/1  "<Primary>"
  Handwheel Angle/1 -> Bus Selector3/1
  GPS Vehicle State/1 -> Bus Selector/1
  PostProc/1 -> Bus Selector1/1
  Software Steering Limit/1 -> Sliding Surface Controller function/5(Handwheel)
  Bus Selector1/1 -> Sliding Surface Controller function/6(d)  "<Composite Steer Angle>"
  Mux/1 -> Named Mux/2
  Sliding Surface Controller function/11(K_control) -> Mux/10

== system UserBlocks/Steering Controller ==
  Handwheel Angle : Inport
  Switches : Inport  Port=2
  Steering Addition : Inport  Port=3
  Ackermann Correction : Subsystem
  Add : Sum
  Bus Selector1 : BusSelector  OutputSignals=Primary
  Bus Selector4 : BusSelector  OutputSignals=Auto-Steer Switch
  D2R : Gain  Gain=pi/180  SaturateOnIntegerOverflow=on  OutDataTypeStr=Inherit: Same as input  ParamDataTypeStr=Inherit: Same as input
  HAL-9000 : Subsystem  mask{enabled=off, maneuver=Chirp, amplitude=5, delay=0, duration=20, startfreq=.5, endfreq=5}
      mask prompts: enabled "Enable HAL-9000 Automated Steering Maneuver System"; maneuver "Steering manuever"; amplitude "Amplitude (deg)"; delay "Delay (sec)"; duration "Duration (sec)"; startfreq "Initial frequency (Hz)"; endfreq "Final frequency (Hz)"
      mask init:
      | switch(maneuver)
      | 	case 'Step'
      | 		maneuver=1;
      | 	case 'Ramp'
      | 		maneuver=2;
      | 	case 'Chirp'
      | 		maneuver=3;
      | 	case 'Double-step'
      | 		maneuver=4;
      | 	case 'Double chirp'
      | 		maneuver=5;
      | end
      | switch(enabled)
      | 	case 'on'
      | 		enabled=1;
      | 	case 'off'
      | 		enabled=0;
      | end
      mask Callback enabled:
      | if(strcmp(get_param(gcb,'enabled'),'off'))
      | 	set_param(gcb,'MaskEnables',{'on','off','off','off','off','off','off'});
      | else
      | 	set_param(gcb,'MaskEnables',{'on','on','on','on','on','on','on'});
      | end
      mask TypeOptions maneuver: Step | Ramp | Chirp | Double step | Double chirp
      mask Callback maneuver:
      | switch(get_param(gcb,'maneuver'))
      | 	case 'Step'
      | 		set_param(gcb,'MaskVisibilities',{'on','on','on','on','off','off','off'});
      | 	case 'Double step'
      | 		set_param(gcb,'MaskVisibilities',{'on','on','on','on','on','off','off'});
      | 	case 'Ramp'
      | 		set_param(gcb,'MaskVisibilities',{'on','on','on','on','on','off','off'});
      | 	case 'Chirp'
      | 		set_param(gcb,'MaskVisibilities',{'on','on','on','on','on','on','on'});
      | 	case 'Double chirp'
      | 		set_param(gcb,'MaskVisibilities',{'on','on','on','on','on','on','on'});
      | end
  Heavy Filter : DiscreteFilter  Numerator=hal_filter_num  Denominator=hal_filter_den  SampleTime=Ts
  Input Selector : Constant  Value=2
  Multiport Switch : MultiPortSwitch
  Mux1 : Mux  Inputs=2
  Nominal Filter : DiscreteFilter  Numerator=[wc*2*pi*Ts]  Denominator=[1 wc*2*pi*Ts-1]  SampleTime=Ts
  Positive Toe Offset (per wheel) : Constant  Value=0
  Software Steering Limit : Saturate  UpperLimit=steering_limit*sr*pi/180  LowerLimit=-steering_limit*sr*pi/180
  Software Steering Limit1 : Saturate  UpperLimit=steering_limit*pi/180  LowerLimit=-steering_limit*pi/180
  Steering Ratio1 : Gain  Gain=sr  SaturateOnIntegerOverflow=on  OutDataTypeStr=Inherit: Same as input  ParamDataTypeStr=Inherit: Same as input
  Steering Ratio : Gain  Gain=1/sr  SaturateOnIntegerOverflow=on  OutDataTypeStr=Inherit: Same as input  ParamDataTypeStr=Inherit: Same as input
  Subtract : Sum  Inputs=-+
  Sum : Sum  Inputs=++|
  Sum1 : Sum  Inputs=+++
  Switch : Switch  Threshold=0.5
  Steering Angle Commands : Outport
  tag scope: global_HAL_command=global
  wires:
  Add/1 -> Mux1/2
  Subtract/1 -> Mux1/1
  Ackermann Correction/2(R Steer Angle) -> Add/2
  Ackermann Correction/1(L Steer Angle) -> Subtract/2
  Steering Ratio/1 -> Software Steering Limit1/1
  Software Steering Limit1/1 -> Ackermann Correction/1(Ackermann Angle)
  Software Steering Limit/1 -> Sum/1
  Handwheel Angle/1 -> Bus Selector1/1
  Switches/1 -> Bus Selector4/1
  Multiport Switch/1 -> Steering Ratio/1
  Bus Selector4/1 -> HAL-9000/1(Trigger), Switch/2  "<Auto-Steer Switch>"
  Steering Addition/1 -> Steering Ratio1/1
  Bus Selector1/1 -> Nominal Filter/1, Heavy Filter/1  "<Primary>"
  Steering Ratio1/1 -> Sum1/3, Sum/2
  Nominal Filter/1 -> Software Steering Limit/1, Multiport Switch/2, Switch/3
  Sum/1 -> Multiport Switch/3
  Heavy Filter/1 -> Sum1/1
  HAL-9000/1(Offset) -> [global_HAL_command], Sum1/2
  Input Selector/1 -> Multiport Switch/1
  Switch/1 -> Multiport Switch/4
  Sum1/1 -> Switch/1
  Mux1/1 -> Steering Angle Commands/1
  D2R/1 -> Add/1, Subtract/1
  Positive Toe Offset (per wheel)/1 -> D2R/1

== system UserBlocks/TTS Steering Control ==
  note: assuming 1 means use the controller
  States : Inport
  Handwheel : Inport  Port=2
  Switches : Inport  Port=3
  Ackermann Correction : Subsystem
  Bus Selector2 : BusSelector  OutputSignals=Primary
  Bus Selector4 : BusSelector  OutputSignals=Auto-Steer Switch,Fault Switch
  Compute Steering Along Path : Subsystem
  Mux6 : Mux  Inputs=2
  SW Steering Limit : Saturate  UpperLimit=steering_limit*pi/180  LowerLimit=-steering_limit*pi/180
  Subsystem : Subsystem
  Switch : Switch  Criteria=u2 ~= 0
  Steering Command : Outport
  Steering Debug : Outport  Port=2
  wires:
  Compute Steering Along Path/1(delta (rad)) -> Switch/1
  Compute Steering Along Path/2(debug) -> Steering Debug/1
  Bus Selector4/2 -> Switch/2  "<Fault Switch>"
  States/1 -> Compute Steering Along Path/1(States)
  Bus Selector4/1 -> Subsystem/2(Switches)  "<Auto-Steer Switch>"
  Bus Selector2/1 -> Subsystem/1(Handwheel)  "<Primary>"
  Switches/1 -> Compute Steering Along Path/2(Switches), Bus Selector4/1
  Handwheel/1 -> Bus Selector2/1
  Subsystem/1(Steering Output) -> Switch/3
  Switch/1 -> SW Steering Limit/1
  Ackermann Correction/2(R Steer Angle) -> Mux6/2
  Ackermann Correction/1(L Steer Angle) -> Mux6/1
  SW Steering Limit/1 -> Ackermann Correction/1(Ackermann Angle)
  Mux6/1 -> Steering Command/1

== system UserBlocks/Cruise Control/ConvertVolt2Force ==
  VoltDesired : Inport
  TorqueDesired : Outport
  wires:
  VoltDesired/1 -> TorqueDesired/1

== system UserBlocks/Cruise Control/Enable Logic ==
  Cruise Control : Inport
  Brake Pedal : Inport  Port=2
  Delay : Subsystem
  Latch1 : Subsystem  TreatAsAtomicUnit=on
  Logical Operator : Logic  Operator=OR  AllPortsSameDT=off  OutDataTypeStr=float('double')
  Logical Operator1 : Logic  AllPortsSameDT=off  OutDataTypeStr=float('double')
  Logical Operator2 : Logic  Operator=NOT  AllPortsSameDT=off  OutDataTypeStr=float('double')
  Enable : Outport
  wires:
  Latch1/1(Out1) -> Enable/1
  Cruise Control/1 -> Delay/1(In), Logical Operator1/1
  Delay/1(Out) -> Logical Operator/1
  Brake Pedal/1 -> Logical Operator2/1, Logical Operator/2
  Logical Operator/1 -> Latch1/Trigger
  Logical Operator1/1 -> Latch1/1(In1)
  Logical Operator2/1 -> Logical Operator1/2

== system UserBlocks/Cruise Control/Pedal Latch ==
  In1 : Inport
  Trigger : TriggerPort
  Out1 : Outport  InitialOutput=0
  wires:
  In1/1 -> Out1/1

== system UserBlocks/Cruise Control/Speed Latch ==
  In1 : Inport
  Trigger : TriggerPort
  Out1 : Outport  InitialOutput=0
  wires:
  In1/1 -> Out1/1

== system UserBlocks/Diagnostic System/Detection ==
  Filtered Residuals : Inport
  Bus Selector : BusSelector  OutputSignals=Resistance,Motor Constant,Lsa,Rsa,yr,Filtered Gearbox Angle,Steering Angle,Filtered Current Error
  Current Error : Subsystem  mask{thresh=2.5}
      mask prompts: thresh "Threshold"
      mask Display: disp(thresh)
  Gearbox Error : Subsystem  mask{thresh=.045}
      mask prompts: thresh "Threshold"
      mask Display: disp(thresh)
  Motor Constant Error : Subsystem  mask{thresh=.03}
      mask prompts: thresh "Threshold"
      mask Display: disp(thresh)
  Mux : Mux  Inputs=8
  Resistance Error : Subsystem  mask{thresh=.05}
      mask prompts: thresh "Threshold"
      mask Display: disp(thresh)
  Steering Error : Subsystem  mask{thresh=2}
      mask prompts: thresh "Threshold"
      mask Display: disp(thresh)
  Yaw Rate Error A : Subsystem  mask{thresh=.03}
      mask prompts: thresh "Threshold"
      mask Display: disp(thresh)
  Yaw Rate Error B : Subsystem  mask{thresh=.03}
      mask prompts: thresh "Threshold"
      mask Display: disp(thresh)
  Yaw Rate Error C : Subsystem  mask{thresh=.2}
      mask prompts: thresh "Threshold"
      mask Display: disp(thresh)
  Boolean Residuals : Outport
  wires:
  Filtered Residuals/1 -> Bus Selector/1
  Bus Selector/7 -> Steering Error/1(Signal)  "<Steering Angle>"
  Steering Error/1(Exceeds Threshold) -> Mux/7
  Bus Selector/1 -> Resistance Error/1(Signal)  "<Resistance>"
  Resistance Error/1(Exceeds Threshold) -> Mux/1
  Bus Selector/2 -> Motor Constant Error/1(Signal)  "<Motor Constant>"
  Motor Constant Error/1(Exceeds Threshold) -> Mux/2
  Bus Selector/3 -> Yaw Rate Error A/1(Signal)  "<Lsa>"
  Yaw Rate Error A/1(Exceeds Threshold) -> Mux/3
  Bus Selector/4 -> Yaw Rate Error B/1(Signal)  "<Rsa>"
  Yaw Rate Error B/1(Exceeds Threshold) -> Mux/4
  Bus Selector/5 -> Yaw Rate Error C/1(Signal)  "<yr>"
  Yaw Rate Error C/1(Exceeds Threshold) -> Mux/5
  Bus Selector/6 -> Gearbox Error/1(Signal)  "<Filtered Gearbox Angle>"
  Gearbox Error/1(Exceeds Threshold) -> Mux/6
  Mux/1 -> Boolean Residuals/1
  Bus Selector/8 -> Current Error/1(Signal)  "<Filtered Current Error>"
  Current Error/1(Exceeds Threshold) -> Mux/8
